simulink model "PerturbnObserve"  (R2014a)
settings: Solver=ode23tb  StartTime=0.0  StopTime=1  MaxStep=0.1  RelTol=1e-3
PreLoadFcn:
  | Ts = 1e-6;
  | G = 1000;
  | PVCellIsc = 7;
  | PVCellVoc = 0.64;
  | PVCellRs = 0.001;
  | tau = 1e-4;
settings Model: Creator=cosorio  LastModifiedBy=cosorio
settings DataIOCC: LimitDataPoints=off  SignalLoggingSaveFormat=ModelDataLogs  SaveOutput=off  SignalLogging=off  DSMLogging=off  SaveTime=off  OutputTimes=[0]
settings OptimizationCC: InlineParams=on  ExpressionDepthLimit=2147483647
settings DebuggingCC: UnderspecifiedInitializationDetection=Classic  SolverPrmCheckMsg=none  FcnCallInpInsideContextMsg=UseLocalSettings  StateNameClashWarn=warning
settings GRTTargetCC: CombineOutputUpdateFcns=off  GRTInterface=on

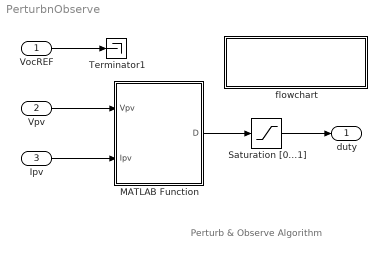
== system PerturbnObserve ==
  note: Perturb & Observe Algorithm
  VocREF : Inport  OutDataTypeStr=double  PortDimensions=1  SampleTime=[0.0001,0]
  Vpv : Inport  Port=2  OutDataTypeStr=double  PortDimensions=1  SampleTime=[0.0001,0]
  Ipv : Inport  Port=3  OutDataTypeStr=double  PortDimensions=1  SampleTime=[0.0001,0]
  MATLAB Function : MATLAB Function  TreatAsAtomicUnit=on
  Saturation [0...1] : Saturate  UpperLimit=1  LowerLimit=0
  Terminator1 : Terminator
  flowchart : Subsystem
      settings: OpenFcn=winopen('PnO.jpg');
      mask Display: disp('Algorithm\nFlowchart')
  duty : Outport  OutDataTypeStr=double  PortDimensions=1  SampleTime=[0.0001,0]
  wires:
  MATLAB Function/1(D) -> Saturation [0...1]/1
  Vpv/1 -> MATLAB Function/1(Vpv)
  Ipv/1 -> MATLAB Function/2(Ipv)
  Saturation [0...1]/1 -> duty/1
  VocREF/1 -> Terminator1/1

== system PerturbnObserve/flowchart ==

== matlab function PerturbnObserve/MATLAB Function ==
  settings: updateMethod=DISCRETE  sampleTime=1e-4
  data: Vpv input; D output; Ipv input
function D = PandO(Vpv,Ipv)
%#codegen
% ************************************************************
% MATLAB implementation of a Perturb and Observe algorithm
% for Maximum Power Point Tracking. This algorithm is designed
% to operate with a buck converter
%
% Created by: Carlos Osorio
% ************************************************************

% Define internal values for the voltage and power as persistent
% variables
persistent Dprev Pprev Vprev

% Initialize the internal values for the voltage and power on the
% first pass
if isempty(Dprev)
    Dprev = 0.7;
    Vprev = 190;
    Pprev = 2000;
end

% Initialize algorithm parameters
deltaD = 0.0025;

% Calculate measured array power
Ppv = Vpv*Ipv;

% Increase or decrease duty cycle based on conditions
if (Ppv-Pprev) ~= 0
    if (Ppv-Pprev) > 0
        if (Vpv-Vprev) > 0
            D = Dprev - deltaD;
        else
            D = Dprev + deltaD;
        end
    else
        if (Vpv-Vprev) > 0
            D = Dprev + deltaD;
        else
            D = Dprev - deltaD;
        end        
    end
else
    D = Dprev;
end

% Update internal values
Dprev = D;
Vprev = Vpv;
Pprev = Ppv;
